simulink model "StateSpaceControl_plusController"  (R2024a)
settings: Solver=VariableStepAuto  StartTime=0.0  StopTime=1  MaxStep=0.2  MinStep=0.0002  RelTol=1e-3
values from neighbouring files (symbols this model uses):
  A = [0, -1; 0, -Rs/Lq]    [StateSpace.m]    (also in untitled.m = [0 1; -100 -5])
  B = [0;1/Lq]    [StateSpace.m]
  C = [0 1]    [StateSpace.m]    (also in untitled.m = [1 0; 0 0]')
  D = [1]    [StateSpace.m]
  Flux = 0.1827    [Parameters.m]    (also in StateSpace.m = 0.192)
  Kd = Kq    [StateSpace.m]
  Kq = place(A,B,pq)    [StateSpace.m]
  Ld = Lq    (= 0.000795)    [StateSpace.m]
  Lq = 0.000795    [StateSpace.m]
  p = 4    [Parameters.m]    (also in StateSpace.m)
  vdc = 560    [StateSpace.m]
libraries: mcbcontrolslib x4, spsControlledVoltageSourceLib x2, spsDCVoltageSourceLib x1, mcbhdlpositiondecoderlib x1, spsPermanentMagnetSynchronousMachineLib x1, spsSVPWMGenerator2LevelLib x1, simulink x1, spsUniversalBridgeLib x1, sps_lib x1
settings Model: Creator=didad  LastModifiedBy=didad

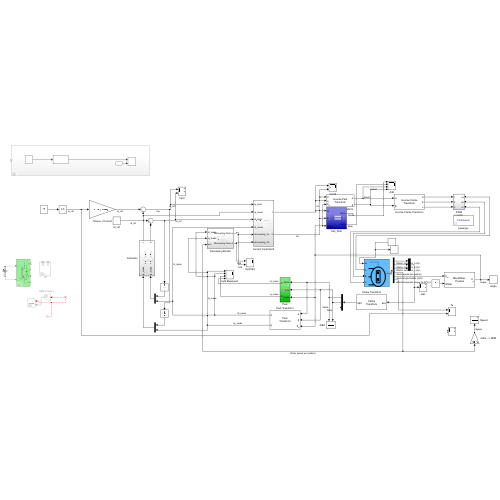
[thumbnail: Simulink's stored preview of the top-level diagram]
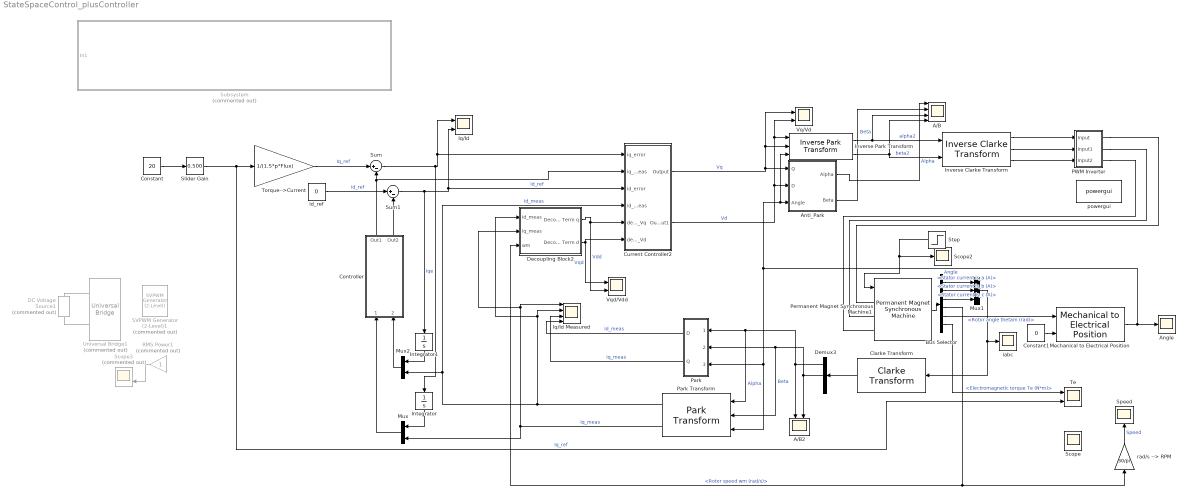
== system StateSpaceControl_plusController ==
  A/B : Scope  NumInputPorts=4
  A/B2 : Scope  NumInputPorts=2
  Angle : Scope
  Anti_Park : Subsystem
  Bus Selector : BusSelector  OutputSignals=Stator current is_a (A),Stator current is_b (A),Stator current is_c (A),Rotor speed wm (rad/s),Rotor angle thetam (rad),Electromagnetic torque Te (N*m)
  Clarke Transform : mcbcontrolslib/Clarke Transform  VariantControl=Variant2  PhaseInput=Three inputs  EnPowerInv=off
      settings: LibrarySourceBlock=mcblib/Controls/Math Transforms/Clarke Transform
  Constant : Constant  Value=20
  Constant1 : Constant  Value=0
  Controller : Subsystem
  Current Controller2 : Subsystem
  DC Voltage Source1 : spsDCVoltageSourceLib/DC Voltage Source  Commented=on  Amplitude=vdc  Measurements=None
  Decoupling Block2 : Subsystem
  Demux3 : Demux  Outputs=3
  Integrator : Integrator
  Integrator1 : Integrator
  Inverse Clarke Transform : mcbcontrolslib/Inverse Clarke Transform  PhaseInput=Two inputs  EnPowerInv=off
      settings: LibrarySourceBlock=mcbhdllib/Controls/Math Transforms/Inverse Clarke Transform
  Inverse Park Transform : mcbcontrolslib/Inverse Park Transform  PhaseInput=Two inputs  AxisAlignment=D-axis  ThetaInput=Electrical position  AngleInput=Radians  N_points=1024
      settings: LibrarySourceBlock=mcbhdllib/Controls/Math Transforms/Inverse Park Transform
  Iq/Id : Scope  NumInputPorts=2
  Iq/Id Measured : Scope  NumInputPorts=4
  Mechanical to Electrical Position : mcbhdlpositiondecoderlib/Mechanical to Electrical Position  PolePairsInputType=Specify via dialog  NrPP=p  selectedRange=Radians  MechOfstInputType=Input port  mechOffsetIn=0  maxAngleIn=2*pi  InputDataType=single  VariantSelect=floating-point
      settings: LibrarySourceBlock=mcbhdllib/Sensor Decoders/Mechanical to Electrical Position
  Mux : Mux  Inputs=2
  Mux1 : Mux  Inputs=3
  Mux2 : Mux  Inputs=2
  PWM Inverter : Subsystem
  Park : Subsystem
  Park Transform : mcbcontrolslib/Park Transform  PhaseInput=Two inputs  AxisAlignment=D-axis  ThetaInput=Electrical position  AngleInput=Radians  N_points=1024
      settings: LibrarySourceBlock=mcblib/Controls/Math Transforms/Park Transform
  Permanent Magnet Synchronous Machine1 : spsPermanentMagnetSynchronousMachineLib/Permanent Magnet Synchronous Machine  NbPhases=3  FluxDistribution=Sinusoidal  RotorType=Round  MechanicalLoad=Speed w  PresetModel="15:  87.75 Nm 560 Vdc 3000 RPM - 97.96 Nm"  ShowDetailedParameters=on  MeasurementBus=off  Resistance=0.05  Inductance=8.5e-3  dqInductances=[0.0007552 0.0008348]  La=0.000795  MachineConstant=Flux linkage established by magnets (V.s)  Flux=0.192  VoltageCst=139.2998  TorqueCst=1.152  Flat=120  Mechanical=[0.011 0.001417 4 0]  PolePairs=4  InitialConditions=[0,0, 0,0]  InitialConditions5ph=[0 0 0 0 0 0]  RefAngle=Aligned with phase A axis (original Park)  IterativeDiscreteModel=Trapezoidal non iterative  TsBlock=-1  TsPowergui=0
  RMS Power1 : Gain  Commented=on
  SVPWM Generator (2-Level)1 : spsSVPWMGenerator2LevelLib/SVPWM Generator (2-Level)  Commented=on  InputType=alpha-beta components  SwitchingPattern=Pattern #1  Fc=fsw  ParUref=[0.8 -30 50]  Ts=0
  Scope : Scope
  Scope2 : Scope
  Scope3 : Scope  Commented=on  NumInputPorts=2
  Slider Gain : simulink/Math Operations/Slider Gain  gain=0.500  low=0  high=2
  Speed : Scope
  Step : Step  Time=0.01  After=10  SampleTime=0
  Subsystem : Subsystem  Commented=on
  Sum : Sum  Inputs=|+-
  Sum1 : Sum  Inputs=|+-
  Te : Scope  NumInputPorts=2
  Torque-->Current : Gain  Gain=1/(1.5*p*Flux)
  Universal Bridge1 : spsUniversalBridgeLib/Universal Bridge  Commented=on  Arms=3  SnubberResistance=1e-5  SnubberCapacitance=inf  Device=IGBT / Diodes  Ron=1e-3  Lon=0  ForwardVoltages="[  0  0  ]"  ForwardVoltage=0  GTOparameters=[ 10e-6 , 20e-6 ]  IGBTparameters=[ 1e-6 , 2e-6 ]  Measurements=None  Measurements_2=None  converterType=Rectifier
  Vq/Vd : Scope  NumInputPorts=2
  Vqd/Vdd : Scope  NumInputPorts=2
  iabc : Scope
  id_ref : Constant  Value=0
  powergui : sps_lib/powergui  Priority=1  SimulationMode=Continuous  SampleTime=50e-6  frequency=60  Iterations=50  frequencyindice=0  Pbase=100e6  ErrMax=1e-4  UnitsV=kV  UnitsW=MW  buscounter=0  FunctionMessages=off  echomessages=off  EnableUseOfTLC=off  CurrentSourceSwitches=off  DisableSnubberDevices=off  DisableRonSwitches=off  DisableVfSwitches=off  DisplayEquations=off  AutomaticDiscreteSolvers=off  SolverType=Tustin/Backward Euler (TBE)  Interpol=off  ExternalGateDelay=off  methode=off  Ts=100  x0status=blocks  SPID=on  SwTol=0  HookPort=off  NonlinearTolerance=1e-4  nMaxIteration=100  ContinueOnMaxIteration=off  RestoreLinks=warning  ResistiveCurrentMeasurement=off  Frange=[0:2:500]  Ylog=off  Xlog=on  ShowGrid=off  save=off  variable=ZData  structure=0  ZoomFFT=off  StartTime=0.0  cycles=1  DisplayStyle=1  fundamental=60  FreqAxis=off  MaxFrequency=1000  frequencyindicesteady=1  RmsSteady=1  display=off
  rad/s --> RPM : Gain  Gain=30/pi
  wires:
  ? -> Scope3/1
  ? -> RMS Power1/1
  Bus Selector/4 -> Decoupling Block2/3(wm), rad/s --> RPM/1  "<Rotor speed wm (rad/s)>"
  Inverse Clarke Transform/2 -> PWM Inverter/2(Input1)
  Mux1/1 -> Clarke Transform/1, iabc/1
  Step/1 -> Permanent Magnet Synchronous Machine1/1, Scope2/1
  Inverse Clarke Transform/3 -> PWM Inverter/3(Input2)
  Bus Selector/3 -> Mux1/3  "<Stator current is_c (A)>"
  Park/1(D) -> Iq/Id Measured/4  "id_meas"
  rad/s --> RPM/1 -> Speed/1  "Speed"
  RMS Power1/1 -> Scope3/2
  Clarke Transform/1 -> Demux3/1
  Current Controller2/1(Output) -> Inverse Park Transform/2, Vq/Vd/1, Anti_Park/1(Q)  "Vq"
  Inverse Clarke Transform/1 -> PWM Inverter/1(Input)
  Bus Selector/6 -> Te/1  "<Electromagnetic torque Te (N*m)>"
  Inverse Park Transform/1 -> A/B/3, Inverse Clarke Transform/1  "alpha2"
  Anti_Park/1(Alpha) -> A/B/1  "Alpha"
  Inverse Park Transform/2 -> A/B/4, Inverse Clarke Transform/2  "beta2"
  Torque-->Current/1 -> Sum/1  "Iq_ref"
  Bus Selector/2 -> Mux1/2  "<Stator current is_b (A)>"
  Constant/1 -> Slider Gain/1
  Demux3/1 -> A/B2/1, Park Transform/1, Park/1(Alpha)  "Alpha"
  Bus Selector/5 -> Mechanical to Electrical Position/1  "<Rotor angle thetam (rad)>"
  Anti_Park/2(Beta) -> A/B/2  "Beta"
  Park Transform/1 -> Mux2/2, Current Controller2/4(id_meas), Iq/Id Measured/2, Decoupling Block2/1(Id_meas)  "Id_meas"
  Permanent Magnet Synchronous Machine1/1 -> Bus Selector/1
  id_ref/1 -> Sum1/1  "id_ref"
  Park/2(Q) -> Iq/Id Measured/3  "iq_meas"
  Sum/1 -> Integrator/1, Iq/Id/1, Current Controller2/1(iq_error)  "Iqe"
  Constant1/1 -> Mechanical to Electrical Position/2
  Bus Selector/1 -> Mux1/1  "<Stator current is_a (A)>"
  Sum1/1 -> Integrator1/1, Iq/Id/2, Current Controller2/3(id_error)  "id_ref"
  Demux3/2 -> A/B2/2, Park Transform/2, Park/2(Beta)  "Beta"
  Slider Gain/1 -> Te/2, Torque-->Current/1  "Iq_ref"
  Park Transform/2 -> Mux/2, Decoupling Block2/2(iq_meas), Iq/Id Measured/1  "Iq_meas"
  Current Controller2/2(Output1) -> Inverse Park Transform/1, Vq/Vd/2, Anti_Park/2(D)  "Vd"
  Decoupling Block2/2(Decoupling Term d) -> Current Controller2/6(decoupling_Vd), Vqd/Vdd/1  "Vqd"
  Decoupling Block2/1(Decoupling Term q) -> Current Controller2/5(decoupling_Vq), Vqd/Vdd/2  "Vdd"
  Mechanical to Electrical Position/1 -> Park Transform/3, Park/3(Angle), Inverse Park Transform/3, Anti_Park/3(Angle), Angle/1  "Angle"
  Controller/1(Out1) -> Current Controller2/2(iq_meas), Sum/2
  Controller/2(Out2) -> Sum1/2
  Mux/1 -> Controller/1(Iq_meas)
  Integrator/1 -> Mux/1
  Integrator1/1 -> Mux2/1
  Mux2/1 -> Controller/2(Id_meas)
  connections:
  PWM Inverter/RConn3 -- Permanent Magnet Synchronous Machine1/LConn3
  Universal Bridge1/RConn1 -- DC Voltage Source1/RConn1
  DC Voltage Source1/LConn1 -- Universal Bridge1/RConn2
  PWM Inverter/RConn1 -- Permanent Magnet Synchronous Machine1/LConn1
  PWM Inverter/RConn2 -- Permanent Magnet Synchronous Machine1/LConn2

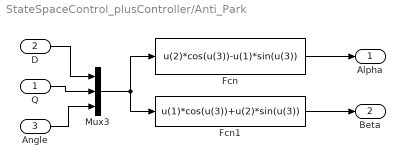
== system StateSpaceControl_plusController/Anti_Park ==
  Q : Inport
  D : Inport  Port=2
  Angle : Inport  Port=3
  Fcn : Fcn  Expr=u(2)*cos(u(3))-u(1)*sin(u(3))
  Fcn1 : Fcn  Expr=u(1)*cos(u(3))+u(2)*sin(u(3))
  Mux3 : Mux  Inputs=3
  Alpha : Outport  VectorParamsAs1DForOutWhenUnconnected=off
  Beta : Outport  Port=2  VectorParamsAs1DForOutWhenUnconnected=off
  wires:
  Angle/1 -> Mux3/3
  Fcn1/1 -> Beta/1
  Mux3/1 -> Fcn1/1, Fcn/1
  Fcn/1 -> Alpha/1
  D/1 -> Mux3/1
  Q/1 -> Mux3/2

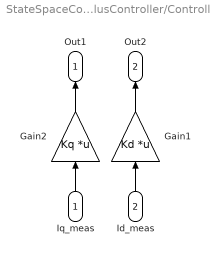
== system StateSpaceControl_plusController/Controller ==
  Iq_meas : Inport
  Id_meas : Inport  Port=2
  Gain1 : Gain  Gain=Kd  Multiplication=Matrix(K*u)
  Gain2 : Gain  Gain=Kq  Multiplication=Matrix(K*u)
  Out1 : Outport
  Out2 : Outport  Port=2
  wires:
  Iq_meas/1 -> Gain2/1
  Id_meas/1 -> Gain1/1
  Gain1/1 -> Out2/1
  Gain2/1 -> Out1/1

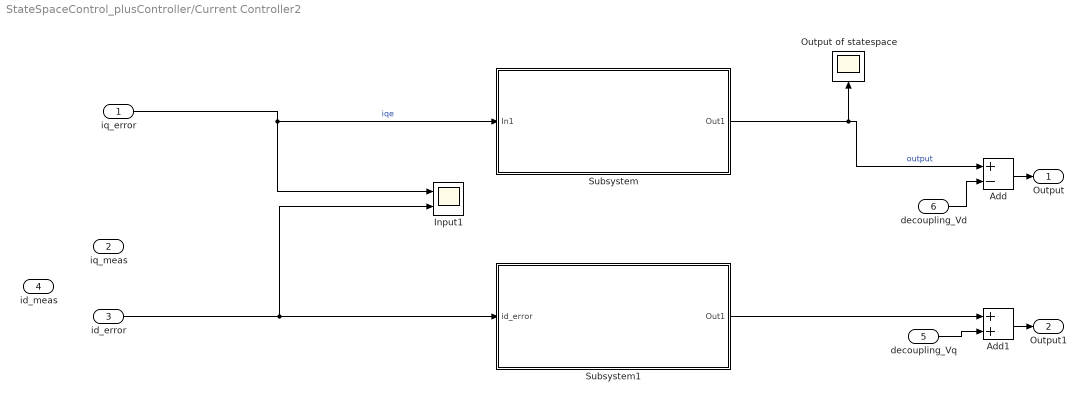
== system StateSpaceControl_plusController/Current Controller2 ==
  iq_error : Inport
  iq_meas : Inport  Port=2
  id_error : Inport  Port=3
  id_meas : Inport  Port=4
  decoupling_Vq : Inport  Port=5
  decoupling_Vd : Inport  Port=6
  Add : Sum  Inputs=+-
  Add1 : Sum
  Input1 : Scope  NumInputPorts=2
  Output of statespace : Scope
  Subsystem : Subsystem
  Subsystem1 : Subsystem
  Output : Outport
  Output1 : Outport  Port=2
  wires:
  Add/1 -> Output/1
  Add1/1 -> Output1/1
  Subsystem1/1(Out1) -> Add1/1
  decoupling_Vq/1 -> Add1/2
  decoupling_Vd/1 -> Add/2
  id_error/1 -> Input1/2, Subsystem1/1(id_error)
  Subsystem/1(Out1) -> Output of statespace/1, Add/1  "output"
  iq_error/1 -> Subsystem/1(In1), Input1/1  "iqe"

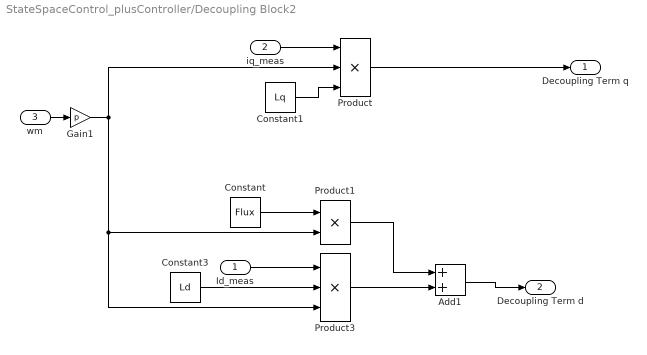
== system StateSpaceControl_plusController/Decoupling Block2 ==
  Id_meas : Inport
  iq_meas : Inport  Port=2
  wm : Inport  Port=3
  Add1 : Sum
  Constant : Constant  Value=Flux
  Constant1 : Constant  Value=Lq
  Constant3 : Constant  Value=Ld
  Gain1 : Gain  Gain=p
  Product : Product  Inputs=3
  Product1 : Product
  Product3 : Product  Inputs=3
  Decoupling Term q : Outport
  Decoupling Term d : Outport  Port=2
  wires:
  Id_meas/1 -> Product3/1
  Gain1/1 -> Product1/2, Product3/3, Product/2
  Constant1/1 -> Product/3
  iq_meas/1 -> Product/1
  Constant3/1 -> Product3/2
  wm/1 -> Gain1/1
  Product/1 -> Decoupling Term q/1
  Product3/1 -> Add1/2
  Constant/1 -> Product1/1
  Product1/1 -> Add1/1
  Add1/1 -> Decoupling Term d/1

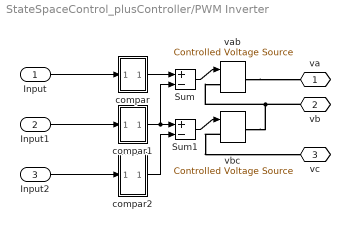
== system StateSpaceControl_plusController/PWM Inverter ==
  Input : Inport
  Input1 : Inport  Port=2
  Input2 : Inport  Port=3
  Sum : Sum  Inputs=+-  InputSameDT=on  SaturateOnIntegerOverflow=on  OutDataTypeStr=Inherit: Same as first input
  Sum1 : Sum  Inputs=+-  InputSameDT=on  SaturateOnIntegerOverflow=on  OutDataTypeStr=Inherit: Same as first input
  compar : Subsystem
  compar1 : Subsystem
  compar2 : Subsystem
  vab : spsControlledVoltageSourceLib/Controlled Voltage Source  Description=source block  Initialize=on  Source_Type=AC  Amplitude=0  Phase=0  Frequency=0  Measurements=None
      settings: AttributesFormatString=\n
  vbc : spsControlledVoltageSourceLib/Controlled Voltage Source  Description=source block  Initialize=on  Source_Type=AC  Amplitude=0  Phase=0  Frequency=0  Measurements=None
      settings: AttributesFormatString=\n
  va : PMIOPort  Side=Right
  vb : PMIOPort  Port=2  Side=Right
  vc : PMIOPort  Port=3  Side=Right
  wires:
  compar/1(va) -> Sum/1
  compar1/1(vb) -> Sum/2, Sum1/1
  compar2/1(vc) -> Sum1/2
  Sum/1 -> vab/1
  Sum1/1 -> vbc/1
  Input/1 -> compar/1(ia)
  Input1/1 -> compar1/1(ib)
  Input2/1 -> compar2/1(ic)
  connections:
  vab/RConn1 -- va/RConn1
  vb/RConn1 -- vab/LConn1 -- vbc/RConn1
  vbc/LConn1 -- vc/RConn1

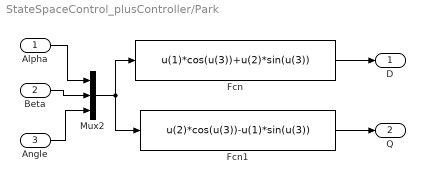
== system StateSpaceControl_plusController/Park ==
  Alpha : Inport
  Beta : Inport  Port=2
  Angle : Inport  Port=3
  Fcn : Fcn  Expr=u(1)*cos(u(3))+u(2)*sin(u(3))
  Fcn1 : Fcn  Expr=u(2)*cos(u(3))-u(1)*sin(u(3))
  Mux2 : Mux  Inputs=3
  D : Outport  VectorParamsAs1DForOutWhenUnconnected=off
  Q : Outport  Port=2  VectorParamsAs1DForOutWhenUnconnected=off
  wires:
  Beta/1 -> Mux2/2
  Mux2/1 -> Fcn1/1, Fcn/1
  Angle/1 -> Mux2/3
  Alpha/1 -> Mux2/1
  Fcn1/1 -> Q/1
  Fcn/1 -> D/1

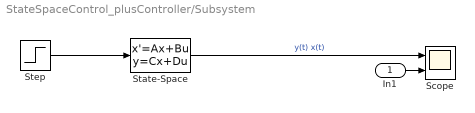
== system StateSpaceControl_plusController/Subsystem ==
  In1 : Inport
  Scope : Scope  NumInputPorts=2
  State-Space : StateSpace  A=A  B=B  C=C  D=D  InitialCondition=0
  Step : Step  SampleTime=0
  wires:
  State-Space/1 -> Scope/1  "y(t) x(t)"
  Step/1 -> State-Space/1
  In1/1 -> Scope/2

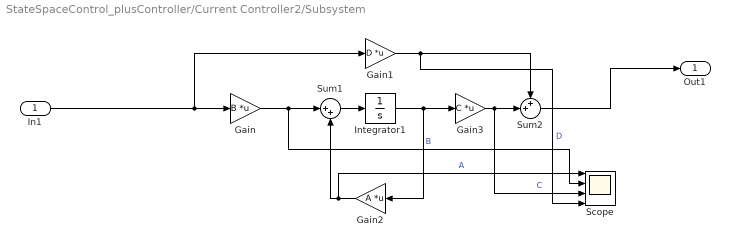
== system StateSpaceControl_plusController/Current Controller2/Subsystem ==
  In1 : Inport
  Gain : Gain  Gain=B  Multiplication=Matrix(K*u)
  Gain1 : Gain  Gain=D  Multiplication=Matrix(K*u)
  Gain2 : Gain  Gain=A  Multiplication=Matrix(K*u)
  Gain3 : Gain  Gain=C  Multiplication=Matrix(K*u)
  Integrator1 : Integrator
  Scope : Scope  NumInputPorts=4
  Sum1 : Sum  Inputs=|++
  Sum2 : Sum  Inputs=++|
  Out1 : Outport
  wires:
  Sum1/1 -> Integrator1/1
  Integrator1/1 -> Gain2/1, Gain3/1
  Gain2/1 -> Scope/1, Sum1/2  "A"
  Gain1/1 -> Scope/4, Sum2/1  "D"
  Gain/1 -> Scope/2, Sum1/1  "B"
  In1/1 -> Gain1/1, Gain/1
  Gain3/1 -> Scope/3, Sum2/2  "C"
  Sum2/1 -> Out1/1

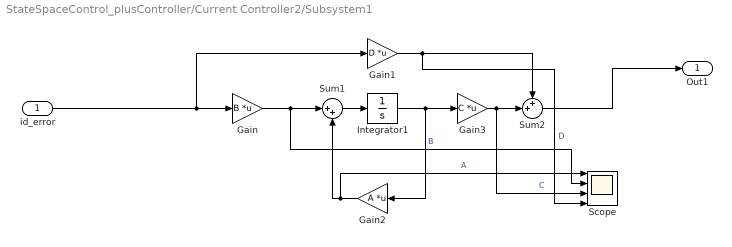
== system StateSpaceControl_plusController/Current Controller2/Subsystem1 ==
  id_error : Inport
  Gain : Gain  Gain=B  Multiplication=Matrix(K*u)
  Gain1 : Gain  Gain=D  Multiplication=Matrix(K*u)
  Gain2 : Gain  Gain=A  Multiplication=Matrix(K*u)
  Gain3 : Gain  Gain=C  Multiplication=Matrix(K*u)
  Integrator1 : Integrator
  Scope : Scope  NumInputPorts=4
  Sum1 : Sum  Inputs=|++
  Sum2 : Sum  Inputs=++|
  Out1 : Outport
  wires:
  Sum1/1 -> Integrator1/1
  Integrator1/1 -> Gain2/1, Gain3/1
  Gain2/1 -> Scope/1, Sum1/2  "A"
  Gain1/1 -> Scope/4, Sum2/1  "D"
  Gain/1 -> Scope/2, Sum1/1  "B"
  id_error/1 -> Gain1/1, Gain/1
  Gain3/1 -> Scope/3, Sum2/2  "C"
  Sum2/1 -> Out1/1

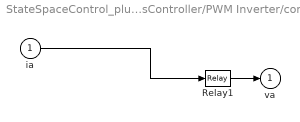
== system StateSpaceControl_plusController/PWM Inverter/compar ==
  ia : Inport
  Relay1 : Relay  OnSwitchValue=0.05  OffSwitchValue=-0.05  OnOutputValue=155  OffOutputValue=-155
  va : Outport  InitialOutput=0  VectorParamsAs1DForOutWhenUnconnected=off
  wires:
  ia/1 -> Relay1/1
  Relay1/1 -> va/1

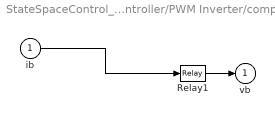
== system StateSpaceControl_plusController/PWM Inverter/compar1 ==
  ib : Inport
  Relay1 : Relay  OnSwitchValue=0.05  OffSwitchValue=-0.05  OnOutputValue=155  OffOutputValue=-155
  vb : Outport  InitialOutput=0  VectorParamsAs1DForOutWhenUnconnected=off
  wires:
  ib/1 -> Relay1/1
  Relay1/1 -> vb/1

== system StateSpaceControl_plusController/PWM Inverter/compar2 ==
  ic : Inport
  Relay1 : Relay  OnSwitchValue=0.05  OffSwitchValue=-0.05  OnOutputValue=155  OffOutputValue=-155
  vc : Outport  InitialOutput=0  VectorParamsAs1DForOutWhenUnconnected=off
  wires:
  ic/1 -> Relay1/1
  Relay1/1 -> vc/1
